simulink model "esn_CPcontrol2"  (R2023a)
settings: Solver=VariableStepAuto  StartTime=0.0  StopTime=stoptime  RelTol=1e-3
values from neighbouring files (symbols this model uses):
  X = esn.train_reservoirReadoutWashed    [ESN_trainbysim.m]
  Y = esn.train_reservoirTargetWashed{i}    [ESN_trainbysim.m]
undefined symbols (not defined in the file or in its folder): arm_radius, arm_radius_previus, cardepth, carlength, carrho, carwidth, esn, ini_theta_p, ini_thetadot_p, ini_x_c, ini_xdot_c, K, pendepth, penlength, penrho, penwidth, spring_position_scale, t_switch, Z
libraries: sm_lib x11, nesl_utility x4
settings Model: Creator=fy264  LastModifiedBy=fy264
settings OptimizationCC: ReuseModelBlockBuffer=off
settings DebuggingCC: AlgebraicLoopMsg=none  ArtificialAlgebraicLoopMsg=none

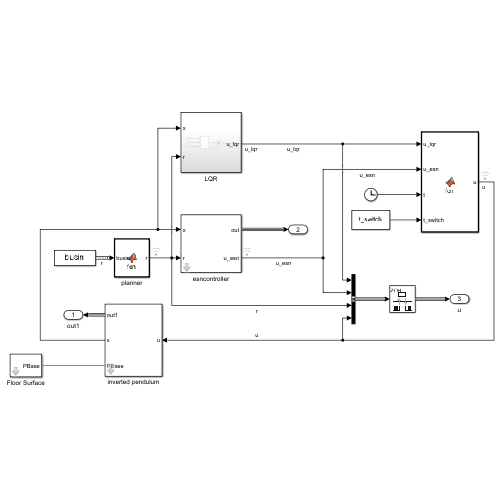
[thumbnail: Simulink's stored preview of the top-level diagram]
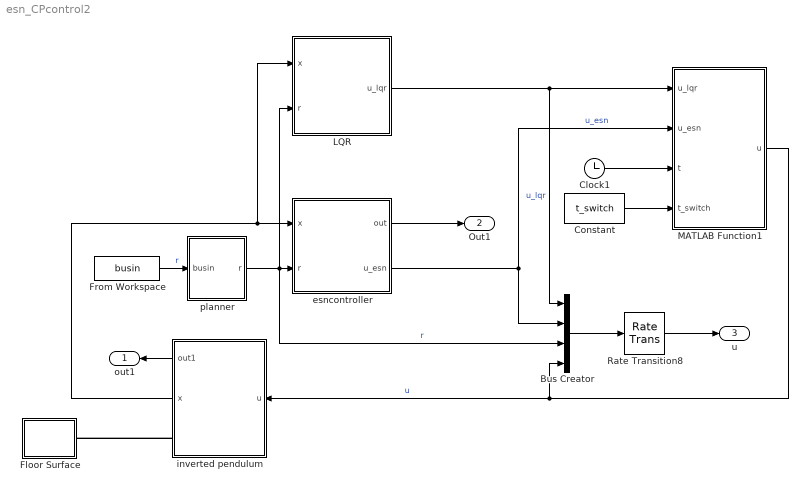
== system esn_CPcontrol2 ==
  Bus Creator : BusCreator  Inputs=4
  Clock1 : Clock
  Constant : Constant  Value=t_switch  VectorParams1D=off
  Floor Surface : Subsystem  mask{length=0.5, width=0.5}
      mask prompts: length "grid length [m]"; width "grid width [m]"
  From Workspace : FromWorkspace  VariableName=busin  OutDataTypeStr=Bus: SinusoidBus
  LQR : Subsystem
  MATLAB Function1 : MATLAB Function  TreatAsAtomicUnit=on
  Rate Transition8 : RateTransition  OutPortSampleTime=esn.timestep
  esncontroller : Subsystem  mask{Nr=esn.Nr, tau=esn.tau, Win=esn.Win, Wb=esn.Wb, Wr=esn.Wr, Wout=esn.Wout{1}, sizeinput=esn.sizeinput, nodenuminput=esn.nodenuminput, timestep=esn.timestep, ini_S=esn.initialstate, delaylen=esn.delaylen, delaynorm=esn.delaynorm, normmethod=esn.normmethod, ifxnorm=esn.ifxnorm, xnorm=esn.xnorm}
  inverted pendulum : Subsystem  mask{carrho=carrho, penrho=penrho, carlength=carlength, carwidth=carwidth, cardepth=cardepth, penlength=penlength, penwidth=penwidth, pendepth=pendepth, ini_x_c=ini_x_c, ini_xdot_c=ini_xdot_c, ini_theta_p=ini_theta_p, ini_thetadot_p=ini_thetadot_p}
  planner : MATLAB Function  TreatAsAtomicUnit=on
  out1 : Outport
  Out1 : Outport  Port=2
  u : Outport  Port=3
  wires:
  From Workspace/1 -> planner/1(busin)  "r"
  inverted pendulum/1(out1) -> out1/1
  inverted pendulum/2(x) -> LQR/1(x), esncontroller/1(x)
  esncontroller/1(out) -> Out1/1
  esncontroller/2(u_esn) -> Bus Creator/2, MATLAB Function1/2(u_esn)  "u_esn"
  Constant/1 -> MATLAB Function1/4(t_switch)
  LQR/1(u_lqr) -> Bus Creator/1, MATLAB Function1/1(u_lqr)  "u_lqr"
  Clock1/1 -> MATLAB Function1/3(t)
  MATLAB Function1/1(u) -> Bus Creator/4, inverted pendulum/1(u)  "u"
  Bus Creator/1 -> Rate Transition8/1
  Rate Transition8/1 -> u/1
  planner/1(r) -> LQR/2(r), esncontroller/2(r), Bus Creator/3  "r"
  connections:
  inverted pendulum/RConn1 -- Floor Surface/RConn1

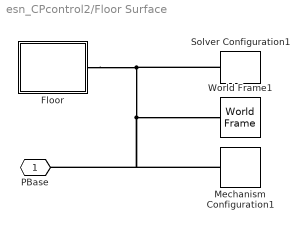
== system esn_CPcontrol2/Floor Surface ==
  Floor : Subsystem
  Mechanism Configuration1 : sm_lib/Utilities/Mechanism Configuration  UniformGravity=Constant  GravityVector=[0 0 -9.80665]  GravityVectorUnits=m/s^2  LinearizationDelta=0.001  JointModeTransitionNonlinearIterations=2
  Solver Configuration1 : nesl_utility/Solver Configuration  PhysicalDomain=network_engine_domain  SubClassName=solver  LeftPortType=input  RightPortType=generic  Tones=[]  Harmonics=[]  SimulateNoise=off  Profile=off  UseLocalSampling=off  EnableSwitchedLinearOptims=on  FrequencyDomain=off  UseCCode=off  RelTol=0.001  AbsTol=1e-06  MinStep=1e-09  ToWorkspace=off  RevertToSquareIcSolve=off  NumHomotopyIterations=100  PhasorMode=off  PhasorModeNumHarmonics=1  ConsistencySolver=NEWTON_FTOL  IndexReductionMethod=DerivativeReplacement  DoDC=off  ResidualTolerance=1e-09  ConsistencyTolSource=GLOBAL  ConsistencyAbsTol=0.001  ConsistencyRelTol=0.001  ConsistencyTolFactor=0.001  UseLocalSolver=off  LocalSolverChoice=NE_BACKWARD_EULER_ADVANCER  ResolveIndetEquations=on  FunctionEvalNumThread=1  LocalSolverSampleTime=0.0002  DoFixedCost=off  MaxNonlinIter=10  MaxModeIter=2  ComputeImpulses=off  ImpulseIterations=2  LinearAlgebra=Sparse  LinearAlgebraNumThread=0  EquationFormulation=NE_TIME_EF  DelaysMemoryBudget=1024  AutomaticFiltering=off  FilteringTimeConstant=0.001  PartitionStorageMethod=AS_NEEDED  PartitionMemoryBudget=1024  PartitionMethod=FAST
  World Frame1 : sm_lib/Frames and Transforms/World Frame
  PBase : PMIOPort  Side=Right
  connections:
  Floor/RConn1 -- PBase/RConn1 -- Mechanism Configuration1/RConn1 -- World Frame1/RConn1 -- Solver Configuration1/RConn1

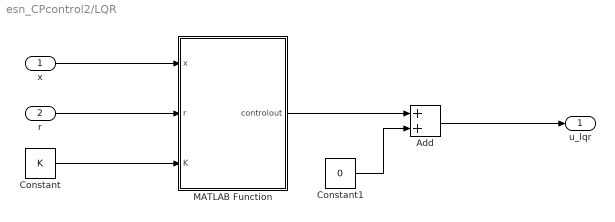
== system esn_CPcontrol2/LQR ==
  x : Inport
  r : Inport  Port=2
  Add : Sum
  Constant : Constant  Value=K  VectorParams1D=off
  Constant1 : Constant  Value=0  VectorParams1D=off
  MATLAB Function : MATLAB Function  TreatAsAtomicUnit=on
  u_lqr : Outport
  wires:
  Constant1/1 -> Add/2
  Add/1 -> u_lqr/1
  Constant/1 -> MATLAB Function/3(K)
  MATLAB Function/1(controlout) -> Add/1
  r/1 -> MATLAB Function/2(r)
  x/1 -> MATLAB Function/1(x)

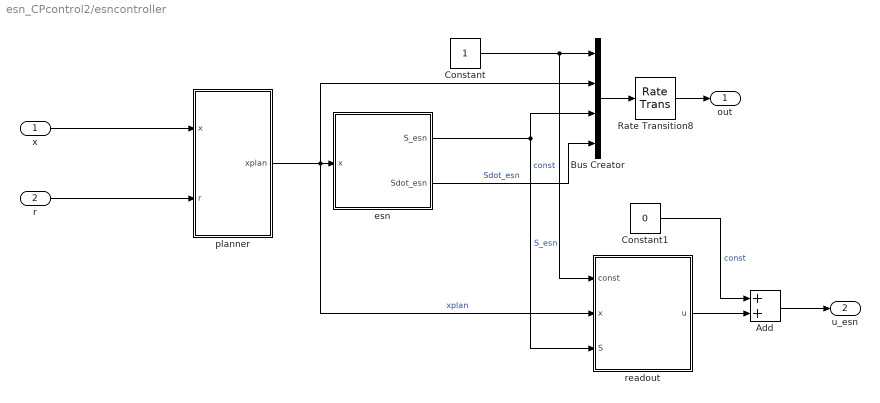
== system esn_CPcontrol2/esncontroller ==
  x : Inport
  r : Inport  Port=2
  Add : Sum
  Bus Creator : BusCreator  Inputs=4
  Constant : Constant
  Constant1 : Constant  Value=0
  Rate Transition8 : RateTransition  OutPortSampleTime=timestep
  esn : Subsystem  mask{Nr=esn.Nr, sizeinput=esn.sizeinput, nodenuminput=esn.nodenuminput, Win=esn.Win, Wr=esn.Wr, Wb=esn.Wb, tau=esn.tau, timestep=esn.timestep, ini_S=esn.initialstate}
  planner : MATLAB Function  TreatAsAtomicUnit=on
  readout : MATLAB Function  TreatAsAtomicUnit=on
  out : Outport
  u_esn : Outport  Port=2
  wires:
  Constant/1 -> readout/1(const), Bus Creator/1  "const"
  Bus Creator/1 -> Rate Transition8/1
  Rate Transition8/1 -> out/1
  planner/1(xplan) -> readout/2(x), Bus Creator/2, esn/1(x)  "xplan"
  esn/2(Sdot_esn) -> Bus Creator/4  "Sdot_esn"
  esn/1(S_esn) -> readout/3(S), Bus Creator/3  "S_esn"
  x/1 -> planner/1(x)
  r/1 -> planner/2(r)
  readout/1(u) -> Add/2
  Add/1 -> u_esn/1
  Constant1/1 -> Add/1  "const"

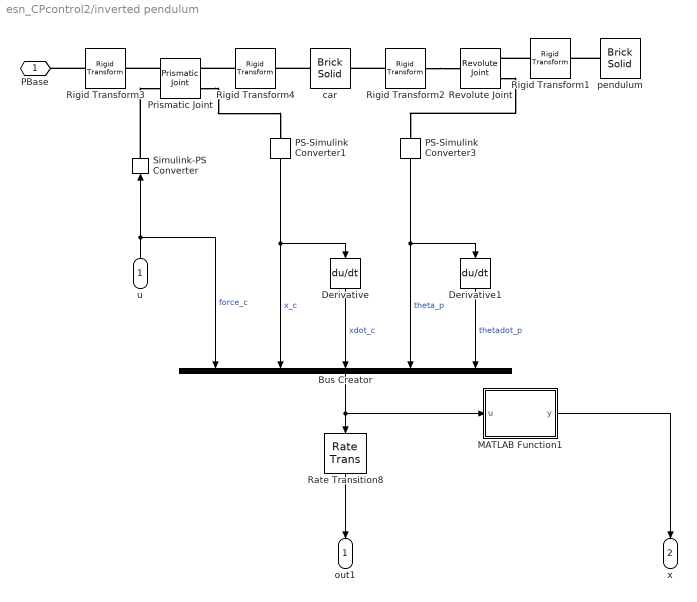
== system esn_CPcontrol2/inverted pendulum ==
  u : Inport
  Bus Creator : BusCreator  Inputs=5
  Derivative : Derivative
  Derivative1 : Derivative
  MATLAB Function1 : MATLAB Function  TreatAsAtomicUnit=on
  PS-Simulink Converter1 : nesl_utility/PS-Simulink Converter  PhysicalDomain=network_engine_domain  SubClassName=ps_output  LeftPortType=input  RightPortType=output  PseudoPeriodic=off  Frequencies=[]  VectorFormat=1-D array  Unit=1  AffineConversion=off
  PS-Simulink Converter3 : nesl_utility/PS-Simulink Converter  PhysicalDomain=network_engine_domain  SubClassName=ps_output  LeftPortType=input  RightPortType=output  PseudoPeriodic=off  Frequencies=[]  VectorFormat=1-D array  Unit=1  AffineConversion=off
  Prismatic Joint : sm_lib/Joints/Prismatic Joint  JointMode=Normal  SenseConstraintForce=off  SenseConstraintForceX=off  SenseConstraintForceY=off  SenseConstraintForceZ=off  SenseConstraintTorque=off  SenseConstraintTorqueX=off  SenseConstraintTorqueY=off  SenseConstraintTorqueZ=off  SenseTotalForce=off  SenseTotalForceX=off  SenseTotalForceY=off  SenseTotalForceZ=off  SenseTotalTorque=off  SenseTotalTorqueX=off  SenseTotalTorqueY=off  SenseTotalTorqueZ=off  CompositeWrenchDir=FollowerOnBase  CompositeWrenchFrame=BaseFrame  EquilibriumPosition=0  EquilibriumPositionUnits=m  SpringStiffness=0  SpringStiffnessUnits=N/m  DampingCoefficient=0  DampingCoefficientUnits=N/(m/s)  TorqueActuationMode=InputTorque  MotionActuationMode=ComputedMotion  SensePosition=on  SenseVelocity=off  SenseAcceleration=off  SenseTorqueForce=off  SenseLowerLimitTorqueForce=off  SenseUpperLimitTorqueForce=off  LowerLimitSpecify=off  LowerLimitBound=-1  LowerLimitBoundUnits=m  LowerLimitStiffness=1e6  LowerLimitStiffnessUnits=N/m  LowerLimitDamping=1e3  LowerLimitDampingUnits=N/(m/s)  LowerLimitTransitionRegionWidth=1e-4  LowerLimitTransitionRegionWidthUnits=m  UpperLimitSpecify=off  UpperLimitBound=1  UpperLimitBoundUnits=m  UpperLimitStiffness=1e6  UpperLimitStiffnessUnits=N/m  UpperLimitDamping=1e3  UpperLimitDampingUnits=N/(m/s)  UpperLimitTransitionRegionWidth=1e-4  UpperLimitTransitionRegionWidthUnits=m  PositionTargetSpecify=on  PositionTargetPriority=Low  PositionTargetValue=ini_x_c  PositionTargetValueUnits=m  VelocityTargetSpecify=on  VelocityTargetPriority=Low  VelocityTargetValue=ini_xdot_c  VelocityTargetValueUnits=m/s
  Rate Transition8 : RateTransition  OutPortSampleTime=0.01
  Revolute Joint : sm_lib/Joints/Revolute Joint  JointMode=Normal  SenseConstraintForce=off  SenseConstraintForceX=off  SenseConstraintForceY=off  SenseConstraintForceZ=off  SenseConstraintTorque=off  SenseConstraintTorqueX=off  SenseConstraintTorqueY=off  SenseConstraintTorqueZ=off  SenseTotalForce=off  SenseTotalForceX=off  SenseTotalForceY=off  SenseTotalForceZ=off  SenseTotalTorque=off  SenseTotalTorqueX=off  SenseTotalTorqueY=off  SenseTotalTorqueZ=off  CompositeWrenchDir=FollowerOnBase  CompositeWrenchFrame=BaseFrame  EquilibriumPosition=0  EquilibriumPositionUnits=deg  SpringStiffness=0  SpringStiffnessUnits=N*m/deg  DampingCoefficient=0  DampingCoefficientUnits=N*m/(deg/s)  TorqueActuationMode=NoTorque  MotionActuationMode=ComputedMotion  SensePosition=on  SenseVelocity=off  SenseAcceleration=off  SenseTorqueForce=off  SenseLowerLimitTorqueForce=off  SenseUpperLimitTorqueForce=off  LowerLimitSpecify=off  LowerLimitBound=-90  LowerLimitBoundUnits=deg  LowerLimitStiffness=1e4  LowerLimitStiffnessUnits=N*m/deg  LowerLimitDamping=10  LowerLimitDampingUnits=N*m/(deg/s)  LowerLimitTransitionRegionWidth=0.1  LowerLimitTransitionRegionWidthUnits=deg  UpperLimitSpecify=off  UpperLimitBound=90  UpperLimitBoundUnits=deg  UpperLimitStiffness=1e4  UpperLimitStiffnessUnits=N*m/deg  UpperLimitDamping=10  UpperLimitDampingUnits=N*m/(deg/s)  UpperLimitTransitionRegionWidth=0.1  UpperLimitTransitionRegionWidthUnits=deg  PositionTargetSpecify=on  PositionTargetPriority=Low  PositionTargetValue=ini_theta_p  PositionTargetValueUnits=rad  VelocityTargetSpecify=on  VelocityTargetPriority=Low  VelocityTargetValue=ini_thetadot_p  VelocityTargetValueUnits=rad/s
  Rigid Transform1 : sm_lib/Frames and Transforms/Rigid Transform  TranslationMethod=None  TranslationStandardOffset=0  TranslationStandardOffsetUnits=m  TranslationStandardAxis=+Z  TranslationCartesianOffset=[arm_radius*spring_position_scale 0 0]  TranslationCartesianOffsetUnits=m  TranslationROffset=arm_radius_previus*spring_position_scale  TranslationROffsetUnits=m  TranslationZOffset=0  TranslationZOffsetUnits=m  TranslationThetaOffset=theta  TranslationThetaOffsetUnits=deg  RotationMethod=AlignedAxes  RotationAngleUnits=deg  RotationStandardAxis=+Z  RotationAngle=180  RotationArbitraryAxis=[0 0 1]  FollAlignAxisA=+X  BaseAlignAxisA=+X  FollAlignAxisB=-Z  BaseAlignAxisB=+Y  RotationSequenceAxes=FollowerAxes  RotationSequence=XYX  RotationSequenceAngles=[0 0 0]  RotationSequenceAnglesUnits=deg  RotationMatrix=[1 0 0; 0 1 0; 0 0 1]  Quaternion=[1 0 0 0]
  Rigid Transform2 : sm_lib/Frames and Transforms/Rigid Transform  TranslationMethod=None  TranslationStandardOffset=0  TranslationStandardOffsetUnits=m  TranslationStandardAxis=+Z  TranslationCartesianOffset=[arm_radius*spring_position_scale 0 0]  TranslationCartesianOffsetUnits=m  TranslationROffset=arm_radius_previus*spring_position_scale  TranslationROffsetUnits=m  TranslationZOffset=0  TranslationZOffsetUnits=m  TranslationThetaOffset=theta  TranslationThetaOffsetUnits=deg  RotationMethod=AlignedAxes  RotationAngleUnits=deg  RotationStandardAxis=+Z  RotationAngle=180  RotationArbitraryAxis=[0 0 1]  FollAlignAxisA=+X  BaseAlignAxisA=+X  FollAlignAxisB=+Y  BaseAlignAxisB=-Z  RotationSequenceAxes=FollowerAxes  RotationSequence=XYX  RotationSequenceAngles=[0 0 0]  RotationSequenceAnglesUnits=deg  RotationMatrix=[1 0 0; 0 1 0; 0 0 1]  Quaternion=[1 0 0 0]
  Rigid Transform3 : sm_lib/Frames and Transforms/Rigid Transform  TranslationMethod=None  TranslationStandardOffset=0  TranslationStandardOffsetUnits=m  TranslationStandardAxis=+Z  TranslationCartesianOffset=[arm_radius*spring_position_scale 0 0]  TranslationCartesianOffsetUnits=m  TranslationROffset=arm_radius_previus*spring_position_scale  TranslationROffsetUnits=m  TranslationZOffset=0  TranslationZOffsetUnits=m  TranslationThetaOffset=theta  TranslationThetaOffsetUnits=deg  RotationMethod=AlignedAxes  RotationAngleUnits=deg  RotationStandardAxis=+Z  RotationAngle=180  RotationArbitraryAxis=[0 0 1]  FollAlignAxisA=+X  BaseAlignAxisA=+Y  FollAlignAxisB=+Y  BaseAlignAxisB=+Z  RotationSequenceAxes=FollowerAxes  RotationSequence=XYX  RotationSequenceAngles=[0 0 0]  RotationSequenceAnglesUnits=deg  RotationMatrix=[1 0 0; 0 1 0; 0 0 1]  Quaternion=[1 0 0 0]
  Rigid Transform4 : sm_lib/Frames and Transforms/Rigid Transform  TranslationMethod=None  TranslationStandardOffset=0  TranslationStandardOffsetUnits=m  TranslationStandardAxis=+Z  TranslationCartesianOffset=[arm_radius*spring_position_scale 0 0]  TranslationCartesianOffsetUnits=m  TranslationROffset=arm_radius_previus*spring_position_scale  TranslationROffsetUnits=m  TranslationZOffset=0  TranslationZOffsetUnits=m  TranslationThetaOffset=theta  TranslationThetaOffsetUnits=deg  RotationMethod=AlignedAxes  RotationAngleUnits=deg  RotationStandardAxis=+Z  RotationAngle=180  RotationArbitraryAxis=[0 0 1]  FollAlignAxisA=+Y  BaseAlignAxisA=+X  FollAlignAxisB=+Z  BaseAlignAxisB=+Y  RotationSequenceAxes=FollowerAxes  RotationSequence=XYX  RotationSequenceAngles=[0 0 0]  RotationSequenceAnglesUnits=deg  RotationMatrix=[1 0 0; 0 1 0; 0 0 1]  Quaternion=[1 0 0 0]
  Simulink-PS Converter : nesl_utility/Simulink-PS Converter  PhysicalDomain=network_engine_domain  SubClassName=ps_input  LeftPortType=input  RightPortType=output  PseudoPeriodic=off  Frequencies=[]  NoiseDistribution=none  NoiseParameters=[]  Unit=1  AffineConversion=off  FilteringAndDerivatives=provide  SimscapeFilterOrder=1  InputFilterTimeConstant=0.001  UdotUserProvided=0
  car : sm_lib/Body Elements/Brick Solid  GraphicAmbientColor=[0.15 0.15 0.15 1.0]  BasedOnType=Density  BrickDimensions=[carwidth cardepth carlength]  BrickDimensionsUnits=m  CenterOfMass=[0 0 0]  CenterOfMassUnits=m  GraphicDiffuseColor=[1.0 0.0 0.0]  Density=carrho  DensityUnits=kg/m^3  DoExposeReferenceFrame=on  GraphicEmissiveColor=[0.0 0.0 0.0 1.0]  ExportEntireGeometry=off  SerializedFrames=<Frames><Frame><Id>Frame1</Id><Value><Name>F1</Name><Origin><Source>ReferenceFrame</Source><FeatureName></FeatureName></Origin><PrimaryAxis><DefinedDirection>+Y</DefinedDirection><Source>ReferenceFrame</Source><SourceDirection>+Y</SourceDirection><FeatureName></FeatureName></PrimaryAxis><SecondaryAxis><DefinedDirection>+X</DefinedDirection><Source>ReferenceFrame</Source><SourceDirection>+X</SourceDirection><FeatureName></FeatureName></SecondaryAxis></Value></Frame></Frames>  MarkerShape=Sphere  MarkerSize=10  GraphicType=FromGeometry  InertiaType=CalculateFromGeometry  Mass=1  MassUnits=kg  MomentsOfInertia=[1 1 1]  MomentsOfInertiaUnits=kg*m^2  GraphicOpacity=1.0  ProductsOfInertia=[0 0 0]  ProductsOfInertiaUnits=kg*m^2  GraphicShininess=75  GraphicSpecularColor=[0.5 0.5 0.5 1.0]  GraphicVisPropType=SimpleVisualProperties
  pendulum : sm_lib/Body Elements/Brick Solid  GraphicAmbientColor=[0.15 0.15 0.15 1.0]  BasedOnType=Density  BrickDimensions=[penwidth pendepth penlength]  BrickDimensionsUnits=m  CenterOfMass=[0 0 0]  CenterOfMassUnits=m  GraphicDiffuseColor=[0.0 0.6 1.0]  Density=penrho  DensityUnits=kg/m^3  DoExposeReferenceFrame=off  GraphicEmissiveColor=[0.0 0.0 0.0 1.0]  ExportEntireGeometry=off  SerializedFrames=<Frames><Frame><Id>Frame1</Id><Value><Name>F1</Name><Origin><Source>GeometricFeature</Source><FeatureName>-z surface</FeatureName></Origin><PrimaryAxis><DefinedDirection>+Z</DefinedDirection><Source>ReferenceFrame</Source><SourceDirection>+Z</SourceDirection><FeatureName></FeatureName></PrimaryAxis><SecondaryAxis><DefinedDirection>+X</DefinedDirection><Source>ReferenceFrame</Source><SourceDirection>+X</SourceDirection><FeatureName></FeatureName></SecondaryAxis></Value></Frame></Frames>  MarkerShape=Sphere  MarkerSize=10  GraphicType=FromGeometry  InertiaType=CalculateFromGeometry  Mass=1  MassUnits=kg  MomentsOfInertia=[1 1 1]  MomentsOfInertiaUnits=kg*m^2  GraphicOpacity=1.0  ProductsOfInertia=[0 0 0]  ProductsOfInertiaUnits=kg*m^2  GraphicShininess=75  GraphicSpecularColor=[0.5 0.5 0.5 1.0]  GraphicVisPropType=SimpleVisualProperties
  PBase : PMIOPort  Side=Right
  out1 : Outport
  x : Outport  Port=2
  wires:
  Rate Transition8/1 -> out1/1
  PS-Simulink Converter1/1 -> Derivative/1, Bus Creator/2  "x_c"
  Derivative/1 -> Bus Creator/3  "xdot_c"
  Derivative1/1 -> Bus Creator/5  "thetadot_p"
  u/1 -> Bus Creator/1, Simulink-PS Converter/1  "force_c"
  PS-Simulink Converter3/1 -> Derivative1/1, Bus Creator/4  "theta_p"
  Bus Creator/1 -> MATLAB Function1/1(u), Rate Transition8/1
  MATLAB Function1/1(y) -> x/1
  connections:
  Rigid Transform3/LConn1 -- PBase/RConn1
  Rigid Transform2/LConn1 -- car/LConn1
  Rigid Transform2/RConn1 -- Revolute Joint/LConn1
  pendulum/LConn1 -- Rigid Transform1/RConn1
  Rigid Transform1/LConn1 -- Revolute Joint/RConn1
  car/RConn1 -- Rigid Transform4/RConn1
  Rigid Transform4/LConn1 -- Prismatic Joint/RConn1
  Prismatic Joint/LConn1 -- Rigid Transform3/RConn1
  Prismatic Joint/RConn2 -- PS-Simulink Converter1/LConn1
  Revolute Joint/RConn2 -- PS-Simulink Converter3/LConn1
  Simulink-PS Converter/RConn1 -- Prismatic Joint/LConn2

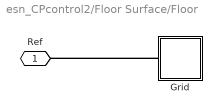
== system esn_CPcontrol2/Floor Surface/Floor ==
  Grid : Subsystem  mask(Grid Lines){grid_origin=[-length -width 0], grid_size=[length width], grid_linewidth=0.001, grid_num_squares=20, grid_color=[0.8 0.8 0.8], grid_opacity=0.8}
      mask prompts: grid_origin "Origin (m)"; grid_size "Arena size (m)"; grid_linewidth "Grid Line Width (m)"; grid_num_squares "Number of Squares"; grid_color "Grid Color [RGB]"; grid_opacity "Grid Opacity (0-1)"
      mask help: Creates grids on 3 planes XZ, YZ, and XZ.
      mask init:
      | mesh_xsec = Extr_Data_Mesh(grid_size(1), grid_size(2), grid_num_squares, grid_num_squares, grid_size(1)/grid_num_squares-grid_linewidth, grid_size(2)/grid_num_squares-grid_linewidth);
  Ref : PMIOPort  Side=Right
  connections:
  Grid/LConn1 -- Ref/RConn1

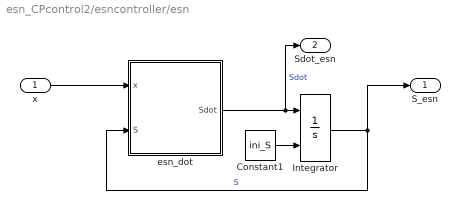
== system esn_CPcontrol2/esncontroller/esn ==
  x : Inport
  Constant1 : Constant  Value=ini_S  VectorParams1D=off
  Integrator : Integrator  InitialConditionSource=external
  esn_dot : MATLAB Function  TreatAsAtomicUnit=on
  S_esn : Outport
  Sdot_esn : Outport  Port=2
  wires:
  esn_dot/1(Sdot) -> Sdot_esn/1, Integrator/1  "Sdot"
  Integrator/1 -> S_esn/1, esn_dot/2(S)  "S"
  Constant1/1 -> Integrator/2
  x/1 -> esn_dot/1(x)

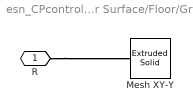
== system esn_CPcontrol2/Floor Surface/Floor/Grid ==
  Mesh XY-Y : sm_lib/Body Elements/Extruded Solid  GraphicAmbientColor=[0.15 0.15 0.15 1.0]  BasedOnType=Density  CenterOfMass=[0 0 0]  CenterOfMassUnits=m  GraphicDiffuseColor=[0.5 0.5 0.5]  ExportConvexHullGeometry=off  ExtrusionCrossSection=mesh_xsec  ExtrusionCrossSectionUnits=m  Density=1000  DensityUnits=kg/(m^3)  DoExposeReferenceFrame=on  GraphicEmissiveColor=[0.0 0.0 0.0 1.0]  ExportEntireGeometry=off  ExtrusionLength=grid_linewidth  ExtrusionLengthUnits=m  ExtrusionType=General  SerializedFrames=<Frames/>  MarkerShape=Sphere  MarkerSize=10  GraphicType=FromGeometry  InertiaType=CalculateFromGeometry  Mass=1  MassUnits=kg  MomentsOfInertia=[1 1 1]  MomentsOfInertiaUnits=kg*m^2  PolygonNumSides=3  GraphicOpacity=1.0  PolygonOuterRadius=1  PolygonOuterRadiusUnits=m  ProductsOfInertia=[0 0 0]  ProductsOfInertiaUnits=kg*m^2  GraphicShininess=75  GraphicSpecularColor=[0.5 0.5 0.5 1.0]  GraphicVisPropType=SimpleVisualProperties
  R : PMIOPort  Side=Left
  connections:
  R/RConn1 -- Mesh XY-Y/RConn1

== matlab function esn_CPcontrol2/planner ==
  data: busin input; r output
function r = fcn(busin)

buscell = struct2cell(busin);

r = [buscell{1}(1);
    buscell{2}(1);
    buscell{3}(1);
    buscell{4}(1)];

end

== matlab function esn_CPcontrol2/esncontroller/esn/esn_dot ==
  data: x input; Sdot output; S input; Nr parameter; sizeinput parameter; nodenuminput parameter; Win parameter; Wr parameter; Wb parameter; tau parameter
function Sdot = fcn(x, S, Nr, sizeinput, nodenuminput, Win, Wr, Wb, tau)

u = zeros(Nr, 1);
for j = 1:sizeinput
    u(j:(j+nodenuminput-1)) = x(j,1);
end

Sdot = (-S + tanh(Win.*u + Wr*S + Wb))/tau;

== matlab function esn_CPcontrol2/esncontroller/readout ==
  data: const input; u output; x input; S input; Wout parameter
function u = fcn(const, x, S, Wout)

readout = [const;x;S];
u = Wout*readout;

end

== matlab function esn_CPcontrol2/inverted pendulum/MATLAB Function1 ==
  data: u input; y output
function y = fcn(u)

y = u(2:end);

== matlab function esn_CPcontrol2/LQR/MATLAB Function ==
  data: x input; r input; controlout output; K input
function controlout = fcn(x, r, K)

% K = [-1.00000000000000	-0.865822552934310	-5.68613442843624	-0.578809286593489];

% r = [r(1);
%     0;
%     0;
%     0;];

controlout = K*(r-x);

end

== matlab function esn_CPcontrol2/MATLAB Function1 ==
  data: u_lqr input; u_esn input; t input; u output; t_switch input
function u = fcn(u_lqr, u_esn, t, t_switch)

if t < t_switch
    u = u_lqr;
else
    u = u_esn;
end

== matlab function esn_CPcontrol2/esncontroller/planner ==
  data: x input; r input; xplan output; delaynorm parameter; normmethod parameter; ifxnorm parameter; xnorm parameter
function xplan = fcn(x, r, delaynorm, normmethod, ifxnorm, xnorm)

if ifxnorm
    x = x./xnorm;
    r = r./xnorm;
end


%planned
dir = r - x;
if vecnorm(dir) == 0
    ref = x;

elseif isnan(delaynorm) || normmethod == 1
    ref = r;

elseif normmethod == 2 || normmethod == 3
    dirnormed = normalize(dir,"norm",2);
    ref = x + dirnormed*min(delaynorm, vecnorm(dir));

elseif normmethod == 4
    dirnormed = normalize(dir,"norm",2);
    ref = x + dirnormed*delaynorm;

else
    ref = r;
end

xplan = [x; ref];

end
